simulink model "observer"  (R2016a)
settings: Solver=VariableStepAuto  StartTime=0.0  StopTime=10  MaxStep=0.01  RelTol=1e-4
values from neighbouring files (symbols this model uses):
  A = [-5.1193e-08 -0.0535; -1.8571 -1.2236]    [Controller_Initial_response.m]    (also in Observer_Initial_response.m; System_behaviour_Stability_Controllability_Observability.m)
  B = [-0.227147; 0.324495]    [Controller_Initial_response.m]    (also in Observer_Initial_response.m; System_behaviour_Stability_Controllability_Observability.m)
  C = [1 0]    [Controller_Initial_response.m]    (also in Observer_Initial_response.m; System_behaviour_Stability_Controllability_Observability.m)
  k = 2    [System_behaviour_Stability_Controllability_Observability.m]
undefined symbols (not defined in the file or in its folder): j
settings Model: Creator=User  LastModifiedBy=User
settings DataIOCC: LimitDataPoints=on  SaveOutput=off  SaveTime=off
settings OptimizationCC: ExpressionDepthLimit=2147483647  LifeSpan=1
settings DebuggingCC: UnderspecifiedInitializationDetection=Classic  MergeDetectMultiDrivingBlocksExec=none  FcnCallInpInsideContextMsg=EnableAllAsWarning  AllowSymbolicDim=off  StateNameClashWarn=warning
settings GRTTargetCC: CombineOutputUpdateFcns=off  GRTInterface=on

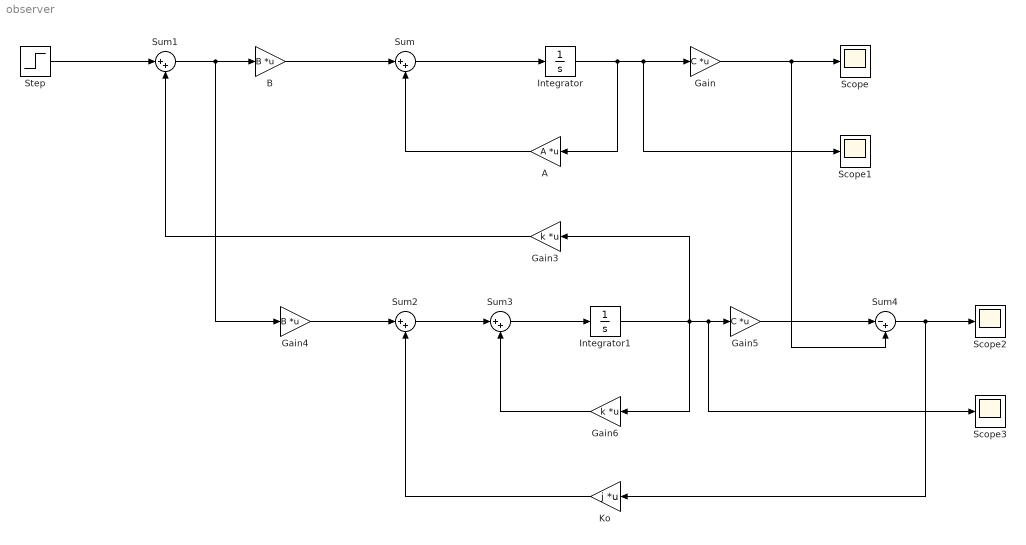
== system observer ==
  A : Gain  Gain=A  Multiplication=Matrix(K*u)
  B : Gain  Gain=B  Multiplication=Matrix(K*u)
  "Gain " : Gain  Gain=C  Multiplication=Matrix(K*u)
  Gain3 : Gain  Gain=k  Multiplication=Matrix(K*u)
  Gain4 : Gain  Gain=B  Multiplication=Matrix(K*u)
  Gain5 : Gain  Gain=C  Multiplication=Matrix(K*u)
  Gain6 : Gain  Gain=k  Multiplication=Matrix(K*u)
  Integrator : Integrator
  Integrator1 : Integrator
  Ko : Gain  Gain=j  Multiplication=Matrix(K*u)
  Scope{,1..3} (4 alike) : Scope
  Step : Step  After=1.3  SampleTime=0.01
  Sum{,1..3} (4 alike) : Sum  Inputs=|++
  Sum4 : Sum  Inputs=|-+
  wires:
  Step/1 -> Sum1/1
  Sum1/1 -> Gain4/1, B/1
  B/1 -> Sum/1
  Sum/1 -> Integrator/1
  Integrator/1 -> A/1, Scope1/1, "Gain "/1
  "Gain "/1 -> Scope/1, Sum4/2
  A/1 -> Sum/2
  Gain3/1 -> Sum1/2
  Gain4/1 -> Sum2/1
  Sum2/1 -> Sum3/1
  Sum3/1 -> Integrator1/1
  Integrator1/1 -> Gain6/1, Gain3/1, Scope3/1, Gain5/1
  Gain5/1 -> Sum4/1
  Sum4/1 -> Ko/1, Scope2/1
  Ko/1 -> Sum2/2
  Gain6/1 -> Sum3/2
